simulink model "SetReset"  (Simulink 8.7)
settings: Solver=FixedStepDiscrete  StartTime=0.0  StopTime=inf  RelTol=1e-3
settings Model: Creator=scaife  LastModifiedBy=hamza  ExtModeAutoUpdateStatusClock=off
settings DataIOCC: SignalLoggingSaveFormat=ModelDataLogs  SignalLoggingName=sigsOut
settings OptimizationCC: InitFltsAndDblsToZero=on
settings DebuggingCC: SaveWithParameterizedLinksMsg=none  SignalResolutionControl=TryResolveAllWithWarning  MultiTaskDSMMsg=warning  MultiTaskCondExecSysMsg=none  StrictBusMsg=None
settings HardwareCC: TargetUnknown=on
settings SFSimCC: SimParseCustomCode=off
settings GRTTargetCC: TargetFcnLib=ansi_tfl_tmw.mat  ModelReferenceCompliant=off  GeneratePreprocessorConditionals=Use local settings  CombineOutputUpdateFcns=off  MatFileLogging=off  GRTInterface=on

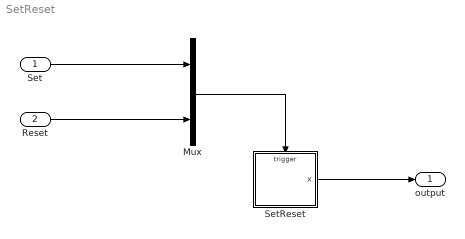
== system SetReset ==
  Set : Inport
  Reset : Inport  Port=2
  Mux : Mux  Inputs=2
  SetReset : Stateflow chart  TreatAsAtomicUnit=on
  output : Outport
  wires:
  Mux/1 -> SetReset/Trigger
  Set/1 -> Mux/1
  Reset/1 -> Mux/2
  SetReset/1(x) -> output/1

== stateflow chart SetReset ==
  state Off/
    en:x=0
  state On/
    en:x=1
  (default) -> Off
  Off -> On : Set
  On -> Off : Reset
  data: x output int32
  events: Set input RISING_EDGE_EVENT; Reset input RISING_EDGE_EVENT
